simulink library "INT_MeUn_VD"  (R2016b)
settings: Solver=VariableStepAuto  StartTime=0.0  StopTime=10.0  RelTol=1e-3
settings Model: Creator=liutao  LastModifiedBy=liutao

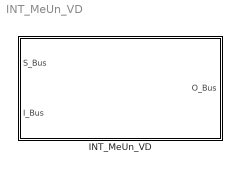
== system INT_MeUn_VD ==
  INT_MeUn_VD : Subsystem

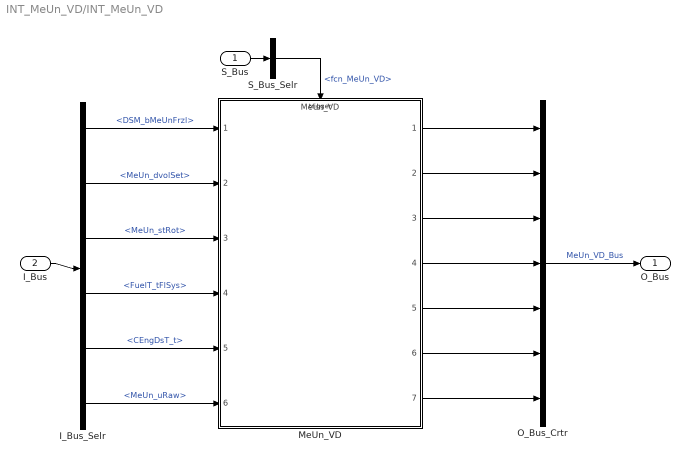
== system INT_MeUn_VD/INT_MeUn_VD ==
  S_Bus : Inport
  I_Bus : Inport  Port=2
  I_Bus_Selr : BusSelector  OutputSignals=DSM_bMeUnFrzl,MeUn_dvolSet,MeUn_stRot,FuelT_tFlSys,CEngDsT_t,MeUn_uRaw
  MeUn_VD : ModelReference  ModelNameDialog=MeUn_VD  SimulationMode=Normal  ModelReferenceVersion=1.27  TriggerPortName=function  TriggerPortTriggerType=function-call  TriggerPortStatesWhenEnabling=held
  O_Bus_Crtr : BusCreator  Inputs=7
  S_Bus_Selr : BusSelector  OutputSignals=fcn_MeUn_VD
  O_Bus : Outport
  wires:
  S_Bus_Selr/1 -> MeUn_VD/Trigger  "<fcn_MeUn_VD>"
  S_Bus/1 -> S_Bus_Selr/1
  I_Bus/1 -> I_Bus_Selr/1
  I_Bus_Selr/1 -> MeUn_VD/1  "<DSM_bMeUnFrzl>"
  I_Bus_Selr/2 -> MeUn_VD/2  "<MeUn_dvolSet>"
  I_Bus_Selr/3 -> MeUn_VD/3  "<MeUn_stRot>"
  I_Bus_Selr/4 -> MeUn_VD/4  "<FuelT_tFlSys>"
  I_Bus_Selr/5 -> MeUn_VD/5  "<CEngDsT_t>"
  I_Bus_Selr/6 -> MeUn_VD/6  "<MeUn_uRaw>"
  O_Bus_Crtr/1 -> O_Bus/1  "MeUn_VD_Bus"
  MeUn_VD/1 -> O_Bus_Crtr/1
  MeUn_VD/2 -> O_Bus_Crtr/2
  MeUn_VD/3 -> O_Bus_Crtr/3
  MeUn_VD/4 -> O_Bus_Crtr/4
  MeUn_VD/5 -> O_Bus_Crtr/5
  MeUn_VD/6 -> O_Bus_Crtr/6
  MeUn_VD/7 -> O_Bus_Crtr/7
